simulink model "FatihErol"  (R2023a)
settings: Solver=VariableStepAuto  StartTime=0.0  StopTime=10.0  RelTol=1e-3
values from neighbouring files (symbols this model uses):
  CD = [0.32 0.16 0.08 0.04 0.02 0.01 0.02 0.04 0.08 0.16 0.32 0.64 ... (13 elements, 13x1)]    [data.mat]
  CL = [-0.6 -0.4 -0.2 0 0.2 0.4 0.6 0.8 1 1.2 1.4 1.6 ... (13 elements, 13x1)]    [data.mat]
  CM = [0.05 0.04 0.03 0.02 0.01 0 -0.01 -0.02 -0.03 -0.04 -0.05 -0.06 ... (13 elements, 13x1)]    [data.mat]
  T = [1 5 5 10 5 5 5 -50 20 50 0]    [data.mat]
libraries: aerolibobsolete x1, aerolibatmos2 x1
settings Model: Creator=Koba  LastModifiedBy=Koba
settings DebuggingCC: UnconnectedInputMsg=warning  UnconnectedOutputMsg=warning  UnconnectedLineMsg=warning
settings ModelReferenceCC: EnableRefExpFcnMdlSchedulingChecks=on
settings RTWCC: DLArmComputeVersion=19.05

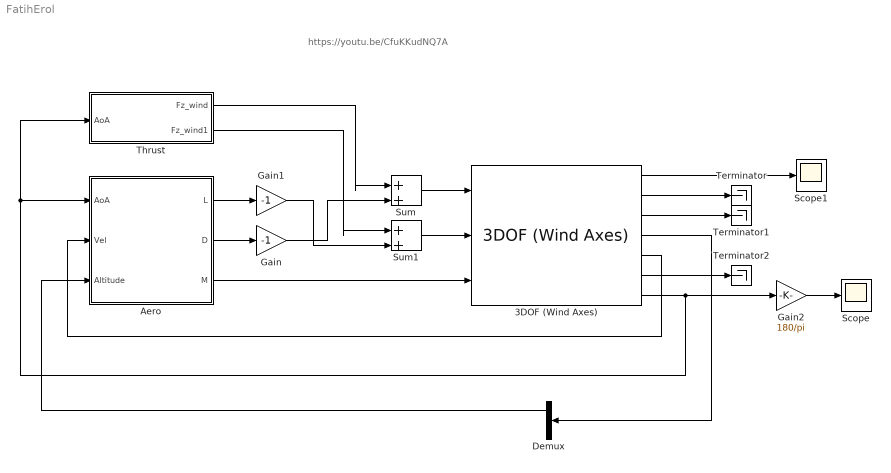
== system FatihErol ==
  note: https://youtu.be/CfuKKudNQ7A
  3DOF (Wind Axes) : aerolibobsolete/3DOF (Wind Axes)  units=Metric (MKS)  mtype=Fixed  V_ini=15  alpha_ini=0  gamma_ini=0  q_ini=0  pos_ini=[0 0]  mass=10  mass_e=0.5  mass_f=3.0  Iyy=1.0  Iyy_e=0.5  Iyy_f=3.0  g_in=Internal  g=9.81  vre_flag=on  abi_flag=off  V_statename=''  alpha_statename=''  gamma_statename=''  q_statename=''  pos_statename=''  mass_statename=''
  Aero : Subsystem
  Demux : Demux  Outputs=2
  Gain : Gain  Gain=-1
  Gain1 : Gain  Gain=-1
  Gain2 : Gain  Gain=180/pi
  Scope : Scope
  Scope1 : Scope
  Sum : Sum  Inputs=|++
  Sum1 : Sum  Inputs=|++
  Terminator : Terminator
  Terminator1 : Terminator
  Terminator2 : Terminator
  Thrust : Subsystem
  wires:
  Sum/1 -> 3DOF (Wind Axes)/1
  Thrust/1(Fz_wind) -> Sum/1
  Gain/1 -> Sum/2
  Sum1/1 -> 3DOF (Wind Axes)/2
  Thrust/2(Fz_wind1) -> Sum1/1
  Gain1/1 -> Sum1/2
  3DOF (Wind Axes)/5 -> Aero/2(Vel)
  3DOF (Wind Axes)/7 -> Gain2/1, Aero/1(AoA), Thrust/1(AoA)
  3DOF (Wind Axes)/2 -> Terminator/1
  3DOF (Wind Axes)/3 -> Terminator1/1
  3DOF (Wind Axes)/6 -> Terminator2/1
  3DOF (Wind Axes)/4 -> Demux/1
  Demux/1 -> Aero/3(Altitude)
  3DOF (Wind Axes)/1 -> Scope1/1
  Gain2/1 -> Scope/1
  Aero/1(L) -> Gain1/1
  Aero/2(D) -> Gain/1
  Aero/3(M) -> 3DOF (Wind Axes)/3

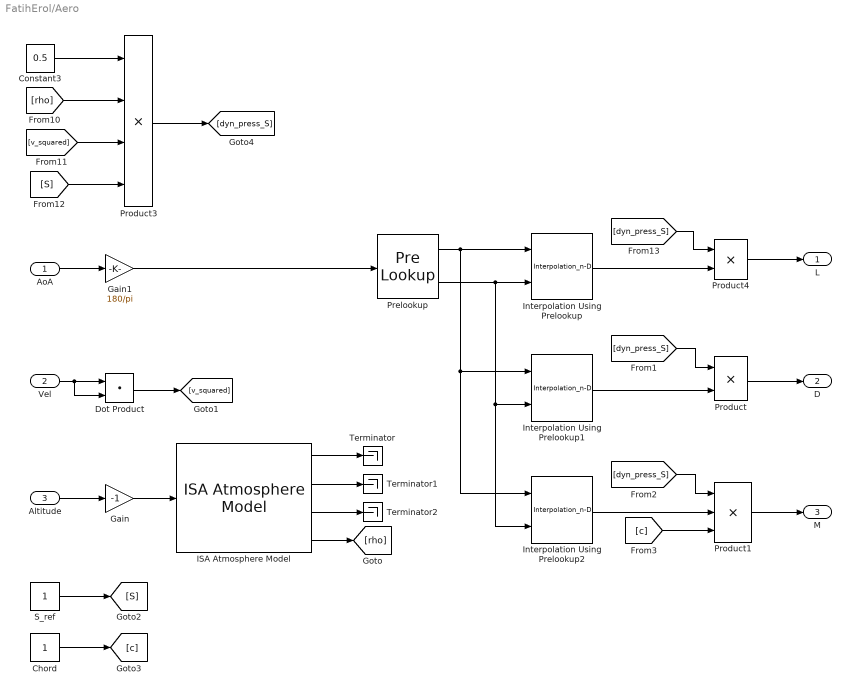
== system FatihErol/Aero ==
  AoA : Inport
  Vel : Inport  Port=2
  Altitude : Inport  Port=3
  Chord : Constant
  Constant3 : Constant  Value=0.5
  Dot Product : DotProduct  OutDataTypeStr=Inherit: Inherit via internal rule
  Gain : Gain  Gain=-1
  Gain1 : Gain  Gain=180/pi
  ISA Atmosphere Model : aerolibatmos2/ISA Atmosphere Model  custom=off  g=9.80665  gamma=1.4  R=287.0531  L=0.0065  h_trop=11000  h_strat=20000  rho0=1.225  P0=101325  T0=288.15  h0=0
  Interpolation Using Prelookup : Interpolation_n-D  NumberOfTableDimensions=1  Table=CL  InternalRulePriority=Speed
      settings: InputPortMap=u0,u1
  Interpolation Using Prelookup1 : Interpolation_n-D  NumberOfTableDimensions=1  Table=CD  InternalRulePriority=Speed
      settings: InputPortMap=u0,u1
  Interpolation Using Prelookup2 : Interpolation_n-D  NumberOfTableDimensions=1  Table=CM  InternalRulePriority=Speed
      settings: InputPortMap=u0,u1
  Prelookup : PreLookup  BreakpointsData=AoA  ExtrapMethod=Linear
  Product : Product
  Product1 : Product  Inputs=3
  Product3 : Product  Inputs=4
  Product4 : Product
  S_ref : Constant
  Terminator : Terminator
  Terminator1 : Terminator
  Terminator2 : Terminator
  L : Outport
  D : Outport  Port=2
  M : Outport  Port=3
  wires:
  Prelookup/1 -> Interpolation Using Prelookup/1, Interpolation Using Prelookup1/1, Interpolation Using Prelookup2/1
  Prelookup/2 -> Interpolation Using Prelookup/2, Interpolation Using Prelookup1/2, Interpolation Using Prelookup2/2
  Altitude/1 -> Gain/1
  Gain/1 -> ISA Atmosphere Model/1
  Vel/1 -> Dot Product/2, Dot Product/1
  AoA/1 -> Gain1/1
  Gain1/1 -> Prelookup/1
  ISA Atmosphere Model/4 -> [rho]
  Dot Product/1 -> [v_squared]
  S_ref/1 -> [S]
  Chord/1 -> [c]
  Interpolation Using Prelookup/1 -> Product4/2
  Interpolation Using Prelookup1/1 -> Product/2
  Interpolation Using Prelookup2/1 -> Product1/2
  ISA Atmosphere Model/1 -> Terminator/1
  ISA Atmosphere Model/2 -> Terminator1/1
  ISA Atmosphere Model/3 -> Terminator2/1
  Constant3/1 -> Product3/1
  [rho] -> Product3/2
  [v_squared] -> Product3/3
  [S] -> Product3/4
  Product3/1 -> [dyn_press_S]
  [dyn_press_S] -> Product4/1
  Product4/1 -> L/1
  [dyn_press_S] -> Product/1
  Product/1 -> D/1
  [dyn_press_S] -> Product1/1
  Product1/1 -> M/1
  [c] -> Product1/3

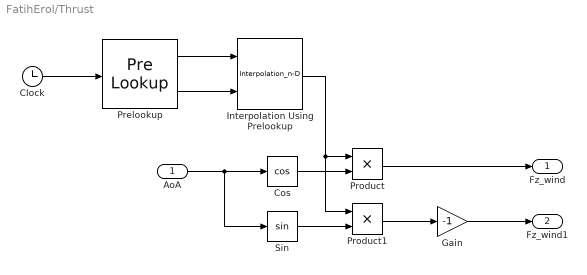
== system FatihErol/Thrust ==
  AoA : Inport
  Clock : Clock
  Cos : Trigonometry  Operator=cos
  Gain : Gain  Gain=-1
  Interpolation Using Prelookup : Interpolation_n-D  NumberOfTableDimensions=1  Table=T  InternalRulePriority=Speed
      settings: InputPortMap=u0,u1
  Prelookup : PreLookup  BreakpointsData=Seconds  ExtrapMethod=Linear
  Product : Product
  Product1 : Product
  Sin : Trigonometry
  Fz_wind : Outport
  Fz_wind1 : Outport  Port=2
  wires:
  Clock/1 -> Prelookup/1
  Prelookup/1 -> Interpolation Using Prelookup/1
  Prelookup/2 -> Interpolation Using Prelookup/2
  AoA/1 -> Sin/1, Cos/1
  Cos/1 -> Product/2
  Sin/1 -> Product1/2
  Product1/1 -> Gain/1
  Gain/1 -> Fz_wind1/1
  Interpolation Using Prelookup/1 -> Product/1, Product1/1
  Product/1 -> Fz_wind/1
